simulink model "blockedrotorbarakat2"  (R2023a)
settings: Solver=VariableStepAuto  StartTime=0.0  StopTime=10.0  RelTol=1e-3
libraries: spsACVoltageSourceLib x3, spsCurrentMeasurementLib x3, spsVoltageMeasurementLib x3, spsRMSLib x2, spsAsynchronousMachineSIUnitsLib x1, spsGroundLib x1, spsPower3phInstantaneousLib x1, sps_lib x1
settings Model: Creator=GTX  LastModifiedBy=GTX

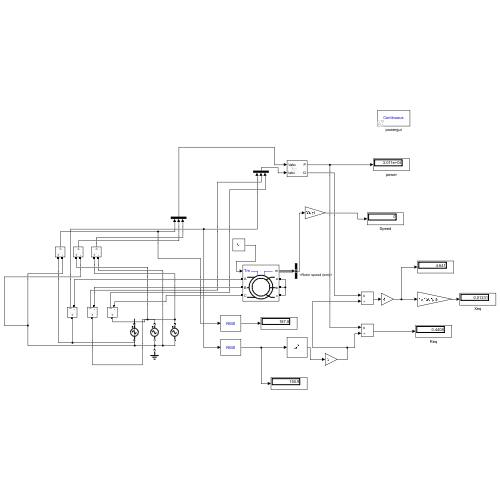
[thumbnail: Simulink's stored preview of the top-level diagram]
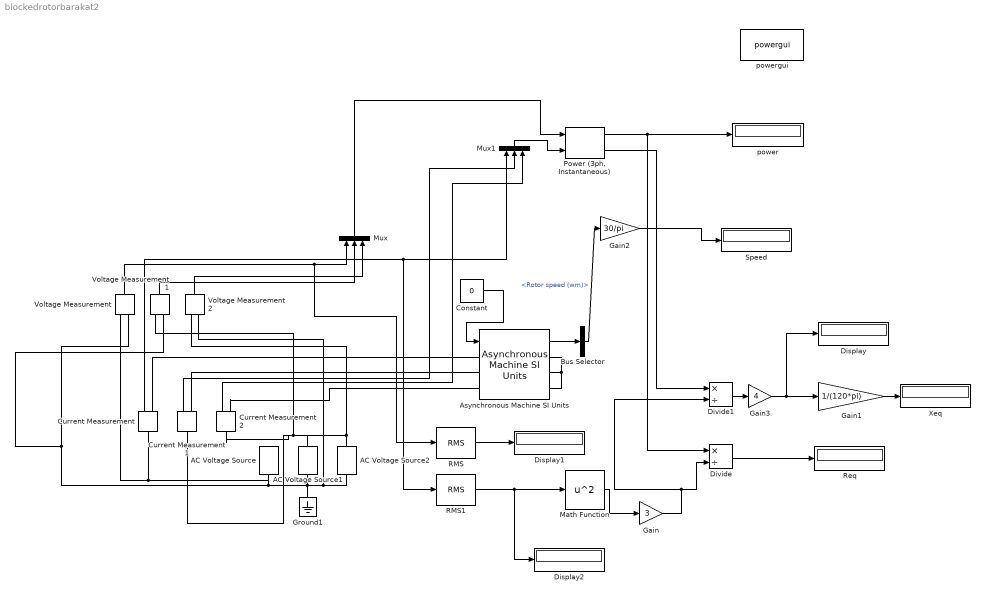
== system blockedrotorbarakat2 ==
  AC Voltage Source : spsACVoltageSourceLib/AC Voltage Source  Amplitude=265.6  Phase=0  Frequency=60  SampleTime=0  Measurements=None  BusType=swing  Pref=10e3  Qref=0  Qmin=-inf  Qmax=+inf
  AC Voltage Source1 : spsACVoltageSourceLib/AC Voltage Source  Amplitude=265.6  Phase=-120  Frequency=60  SampleTime=0  Measurements=None  BusType=swing  Pref=10e3  Qref=0  Qmin=-inf  Qmax=+inf
  AC Voltage Source2 : spsACVoltageSourceLib/AC Voltage Source  Amplitude=265.6  Phase=120  Frequency=60  SampleTime=0  Measurements=None  BusType=swing  Pref=10e3  Qref=0  Qmin=-inf  Qmax=+inf
  Asynchronous Machine SI Units : spsAsynchronousMachineSIUnitsLib/Asynchronous Machine SI Units  RotorType=Wound  PresetModel=No  MechanicalLoad=Torque Tm  ShowDetailedParameters=on  ReferenceFrame=Rotor  Units=SI  MeasurementBus=off  NominalParameters=[18e+03 460 60]  VoltageRatio=1  Stator=[0.2771 0.00170]  Rotor=[0.1771 0.00143]  Cage1=[0.4155 0.002066]  Cage2=[0.4168 0.0003495]  Lm=0.0434  Mechanical=[inf 0.005879 2]  PolePairs=2  InitialConditions=[1 0 0 0 0 0 0 0]  SimulateSaturation=off  Saturation=[14.03593122, 27.81365428, 53.79336849, 72.68890987, 97.98006896, 148.6815601, 215.7428561, 302.9841135, 428.7778367 ; 230, 322, 414, 460, 506, 552, 598, 644, 690]  LoadFlowParameters=1492000  TsPowergui=0  TsBlock=-1  IterativeModel=Trapezoidal non iterative  IterativeDiscreteModel=Trapezoidal non iterative  Pmec=1.492e+006
  Bus Selector : BusSelector  OutputSignals=Mechanical.Rotor speed (wm)
  Constant : Constant  Value=0
  Current Measurement : spsCurrentMeasurementLib/Current Measurement  PhasorSimulation=off  OutputType=Complex  PSBequivalent=0
  Current Measurement1 : spsCurrentMeasurementLib/Current Measurement  PhasorSimulation=off  OutputType=Complex  PSBequivalent=0
  Current Measurement2 : spsCurrentMeasurementLib/Current Measurement  PhasorSimulation=off  OutputType=Complex  PSBequivalent=0
  Display : Display
  Display1 : Display
  Display2 : Display
  Divide : Product  Inputs=*/
  Divide1 : Product  Inputs=*/
  Gain : Gain  Gain=3
  Gain1 : Gain  Gain=1/(120*pi)
  Gain2 : Gain  Gain=30/pi
  Gain3 : Gain  Gain=4
  Ground1 : spsGroundLib/Ground  LConnTagsString=a
  Math Function : Math  Operator=square
  Mux : Mux  Inputs=3
  Mux1 : Mux  Inputs=3
  "Power (3ph, Instantaneous)" : spsPower3phInstantaneousLib/Power (3ph, Instantaneous)
  RMS : spsRMSLib/RMS  TrueRMS=on  Freq=15  RMSInit=120  Ts=0
  RMS1 : spsRMSLib/RMS  TrueRMS=on  Freq=15  RMSInit=120  Ts=0
  Req : Display
  Speed : Display
  Voltage Measurement : spsVoltageMeasurementLib/Voltage Measurement  PhasorSimulation=off  OutputType=Complex  PSBequivalent=0
  Voltage Measurement1 : spsVoltageMeasurementLib/Voltage Measurement  PhasorSimulation=off  OutputType=Complex  PSBequivalent=0
  Voltage Measurement2 : spsVoltageMeasurementLib/Voltage Measurement  PhasorSimulation=off  OutputType=Complex  PSBequivalent=0
  Xeq : Display
  power : Display
  powergui : sps_lib/powergui  Priority=1  SimulationMode=Continuous  SampleTime=50e-6  frequency=60  Iterations=50  frequencyindice=60  Pbase=100e6  ErrMax=1e-4  UnitsV=kV  UnitsW=MW  buscounter=0  FunctionMessages=off  echomessages=off  EnableUseOfTLC=off  CurrentSourceSwitches=off  DisableSnubberDevices=off  DisableRonSwitches=off  DisableVfSwitches=off  DisplayEquations=off  AutomaticDiscreteSolvers=off  SolverType=Tustin/Backward Euler (TBE)  Interpol=off  ExternalGateDelay=off  methode=off  Ts=100  x0status=blocks  SPID=on  SwTol=0  HookPort=off  NonlinearTolerance=1e-4  nMaxIteration=100  ContinueOnMaxIteration=off  RestoreLinks=warning  ResistiveCurrentMeasurement=off  Frange=[0:2:500]  Ylog=off  Xlog=on  ShowGrid=off  save=off  variable=ZData  structure=0  ZoomFFT=off  StartTime=0.0  cycles=1  DisplayStyle=1  fundamental=60  FreqAxis=off  MaxFrequency=1000  frequencyindicesteady=1  RmsSteady=1  display=off
  wires:
  Voltage Measurement/1 -> RMS/1, Mux/1
  Current Measurement2/1 -> Mux1/3
  Current Measurement/1 -> RMS1/1, Mux1/1
  Voltage Measurement2/1 -> Mux/3
  Mux/1 -> "Power (3ph, Instantaneous)"/1
  Mux1/1 -> "Power (3ph, Instantaneous)"/2
  Current Measurement1/1 -> Mux1/2
  Voltage Measurement1/1 -> Mux/2
  "Power (3ph, Instantaneous)"/1 -> Divide/1, power/1
  Constant/1 -> Asynchronous Machine SI Units/1
  Asynchronous Machine SI Units/1 -> Bus Selector/1
  Gain2/1 -> Speed/1
  Bus Selector/1 -> Gain2/1  "<Rotor speed (wm)>"
  Math Function/1 -> Gain/1
  RMS1/1 -> Display2/1, Math Function/1
  Gain/1 -> Divide1/2, Divide/2
  Divide/1 -> Req/1
  "Power (3ph, Instantaneous)"/2 -> Divide1/1
  Divide1/1 -> Gain3/1
  Gain1/1 -> Xeq/1
  Gain3/1 -> Display/1, Gain1/1
  RMS/1 -> Display1/1
  connections:
  Asynchronous Machine SI Units/RConn2 -- Asynchronous Machine SI Units/RConn3 -- Asynchronous Machine SI Units/RConn1
  Voltage Measurement1/LConn1 -- AC Voltage Source1/RConn1 -- Current Measurement1/LConn1
  Current Measurement2/LConn1 -- AC Voltage Source2/RConn1 -- Voltage Measurement2/LConn1
  Ground1/LConn1 -- AC Voltage Source2/LConn1 -- Voltage Measurement2/LConn2 -- Voltage Measurement1/LConn2 -- Voltage Measurement/LConn2 -- AC Voltage Source/LConn1 -- AC Voltage Source1/LConn1
  Voltage Measurement/LConn1 -- AC Voltage Source/RConn1 -- Current Measurement/LConn1
  Current Measurement2/RConn1 -- Asynchronous Machine SI Units/LConn3
  Current Measurement1/RConn1 -- Asynchronous Machine SI Units/LConn2
  Current Measurement/RConn1 -- Asynchronous Machine SI Units/LConn1
